simulink model "controllerBat"  (R2018b)
settings: Solver=VariableStepAuto  StartTime=0.0  StopTime=10.0  RelTol=1e-3
settings Model: Creator=K2  LastModifiedBy=K2

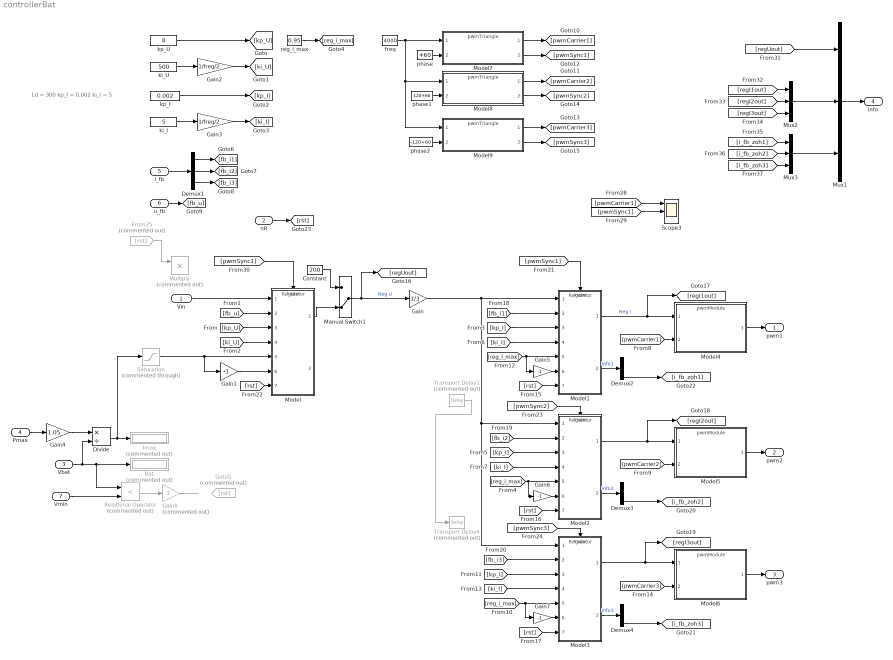
== system controllerBat ==
  note: Ld = 300
      | kp_I = 0.002
      | ki_I = 5
  Vin : Inport
  nR : Inport  Port=2
  Vbat : Inport  Port=3
  Pmax : Inport  Port=4
  i_fb : Inport  Port=5
  u_fb : Inport  Port=6
  Vmin : Inport  Port=7
  Bat : Display  Commented=on
      settings: Format=bank
  Constant : Constant  Value=200
  Demux1 : Demux  Outputs=3
  Demux2 : Demux
  Demux3 : Demux
  Demux4 : Demux
  Divide : Product  Inputs=*/
  From25 : From  Commented=on  GotoTag=rst
  Gain : Gain  Gain=1/3
  Gain{1,5..7} (4 alike) : Gain  Gain=-1
  Gain2 : Gain  Gain=1/freq/2
  Gain3 : Gain  Gain=1/freq/2
  Gain4 : Gain  Gain=1.05
  Gain8 : Gain  Commented=on  OutDataTypeStr=double
  Goto5 : Goto  Commented=on  GotoTag=rst
  Imax : Display  Commented=on
      settings: Format=bank
  Manual Switch1 : ManualSwitch  CurrentSetting=0
  Model{,1..3} (4 alike) : ModelReference  ModelNameDialog=Regulator.slx  SimulationMode=Normal  ModelReferenceVersion=1.46  TriggerPortName=Trigger  TriggerPortTriggerType=either
  Model4 : ModelReference  ModelNameDialog=pwmModule.slx  SimulationMode=Normal  ModelReferenceVersion=1.3
  Model5 : ModelReference  ModelNameDialog=pwmModule.slx  SimulationMode=Normal  ModelReferenceVersion=1.3
  Model6 : ModelReference  ModelNameDialog=pwmModule.slx  SimulationMode=Normal  ModelReferenceVersion=1.3
  Model7 : ModelReference  ModelNameDialog=pwmTriangle.slx  SimulationMode=Normal  ModelReferenceVersion=1.5
  Model8 : ModelReference  ModelNameDialog=pwmTriangle.slx  SimulationMode=Normal  ModelReferenceVersion=1.5
  Model9 : ModelReference  ModelNameDialog=pwmTriangle.slx  SimulationMode=Normal  ModelReferenceVersion=1.5
  Multiply : Product  Commented=on
  Mux1 : Mux  Inputs=3
  Mux2 : Mux  Inputs=3
  Mux3 : Mux  Inputs=3
  Relational Operator : RelationalOperator  Commented=on  Operator=<  OutDataTypeStr=boolean  RndMeth=Simplest
  Saturation : Saturate  Commented=through  UpperLimit=150  LowerLimit=0
  Scope3 : Scope  NumInputPorts=3
  Transport Delay1 : TransportDelay  Commented=on  DelayTime=1/freq/2/3
  Transport Delay4 : TransportDelay  Commented=on  DelayTime=1/freq/2/3
  freq : Constant  Value=4000
  ki_I : Constant  Value=5
  ki_U : Constant  Value=500
  kp_I : Constant  Value=0.002
  kp_U : Constant  Value=8
  phase : Constant  Value=+60
  phase1 : Constant  Value=120+60
  phase2 : Constant  Value=-120+60
  reg_i_max : Constant  Value=0.95
  pwm1 : Outport
  pwm2 : Outport  Port=2
  pwm3 : Outport  Port=3
  info : Outport  Port=4  OutDataTypeStr=double
  wires:
  [pwmSync1] -> Model/Trigger
  Constant/1 -> Manual Switch1/1
  Vbat/1 -> Relational Operator/1, Bat/1, Divide/2
  [reg_i_max] -> Gain7/1, Model3/5
  reg_i_max/1 -> [reg_i_max]
  Model9/2 -> [pwmSync3]
  [pwmSync1] -> Scope3/2
  [pwmSync1] -> Model1/Trigger
  Gain4/1 -> Divide/1
  [ki_I] -> Model3/4
  Divide/1 -> Saturation/1, Imax/1
  [kp_I] -> Model3/3
  freq/1 -> Model8/1, Model9/1, Model7/1
  Model8/2 -> [pwmSync2]
  [pwmCarrier1] -> Scope3/1
  [pwmCarrier2] -> Model5/2
  [ki_U] -> Model/4
  Model4/1 -> pwm1/1
  [pwmSync3] -> Model3/Trigger
  Gain2/1 -> [ki_U]
  [fb_u] -> Model/2
  [kp_U] -> Model/3
  Model9/1 -> [pwmCarrier3]
  Transport Delay1/1 -> Transport Delay4/1
  u_fb/1 -> [fb_u]
  [pwmCarrier3] -> Model6/2
  Pmax/1 -> Gain4/1
  [pwmCarrier1] -> Model4/2
  Model7/2 -> [pwmSync1]
  Gain5/1 -> Model1/6
  Model1/1 -> [regI1out], Model4/1  "Reg I"
  phase/1 -> Model7/2
  [rst] -> Model3/7
  Model3/1 -> [regI3out], Model6/1
  ki_U/1 -> Gain2/1
  [rst] -> Model1/7
  [reg_i_max] -> Gain6/1, Model2/5
  kp_I/1 -> [kp_I]
  [ki_I] -> Model1/4
  Demux1/3 -> [fb_i3]
  Gain7/1 -> Model3/6
  phase2/1 -> Model9/2
  [fb_i2] -> Model2/2
  [kp_I] -> Model1/3
  Model/1 -> Manual Switch1/2
  kp_U/1 -> [kp_U]
  Model8/1 -> [pwmCarrier2]
  i_fb/1 -> Demux1/1
  Gain1/1 -> Model/6
  [ki_I] -> Model2/4
  ki_I/1 -> Gain3/1
  Manual Switch1/1 -> Gain/1, [regUout]  "Reg U"
  [fb_i1] -> Model1/2
  Model7/1 -> [pwmCarrier1]
  [pwmSync2] -> Model2/Trigger
  [rst] -> Model2/7
  phase1/1 -> Model8/2
  Demux1/2 -> [fb_i2]
  [kp_I] -> Model2/3
  Model6/1 -> pwm3/1
  Model2/1 -> Model5/1, [regI2out]
  Gain/1 -> Model3/1, Model2/1, Model1/1
  Gain3/1 -> [ki_I]
  Model5/1 -> pwm2/1
  [fb_i3] -> Model3/2
  Demux1/1 -> [fb_i1]
  [reg_i_max] -> Gain5/1, Model1/5
  Vin/1 -> Model/1
  Gain6/1 -> Model2/6
  Mux3/1 -> Mux1/3
  [i_fb_zoh1] -> Mux3/1
  [i_fb_zoh2] -> Mux3/2
  [i_fb_zoh3] -> Mux3/3
  Mux1/1 -> info/1
  [regI1out] -> Mux2/1
  [regI2out] -> Mux2/2
  [regUout] -> Mux1/1
  [regI3out] -> Mux2/3
  Mux2/1 -> Mux1/2
  Demux2/4 -> [i_fb_zoh1]
  Model1/2 -> Demux2/1  "info1"
  Demux3/4 -> [i_fb_zoh2]
  Model2/2 -> Demux3/1  "info2"
  Demux4/4 -> [i_fb_zoh3]
  Model3/2 -> Demux4/1  "info3"
  Vmin/1 -> Relational Operator/2
  Relational Operator/1 -> Gain8/1
  [rst] -> Model/7
  Gain8/1 -> ?
  From25/1 -> Multiply/1
  Saturation/1 -> Gain1/1, Model/5
  nR/1 -> [rst]
